simulink model "Quad_model"  (R2024b)
settings: Solver=VariableStepAuto  StartTime=0.0  StopTime=50  RelTol=1e-3
model workspace (MATLAB code in the model file):
  | % Quadcopter parameters
  | m = 1.1;            % Mass [kg]
  | ixx = 8.95e-03;     % Moment of inertia (x-axis) [kg.m^2]
  | iyy = 8.95e-03;     % Moment of inertia (y-axis) [kg.m^2]
  | izz = 0.0165;       % Moment of inertia (z-axis) [kg.m^2]
  | g = 9.81;           % Gravitational acceleration [m/s^2]
  | b = 9.60e-06;       % Thrust coefficient [Ns^2/rad^2]
  | d = 1.24e-07;       % Drag coefficient [Ns^2/rad^2]
  | L = 0.25;           % Arm length [m] (converted from 2.50E-01)
  | I = [ixx, 0, 0;
  |     0, iyy, 0;
  |     0, 0, izz];       % the stifness matrix
  | allocation_matrix_1 = [0, 0.5, 0.25, 0.25;
  |                        -0.5, 0, -0.25, 0.25;
  |                         0, -0.5, 0.25, 0.25;
  |                         0.5, 0, -0.25, 0.25];
  | % Compute pseudo-inverse
  | B = [0, -b*L, 0, b*L;
  |      b*L, 0, -b*L, 0;
  |      d, -d, d, -d;
  |      b, b, b, b];
  | A0 = pinv(B);
  | 
  | % Scale columns by max absolute value
  | A_scaled = zeros(size(A0));
  | for j = 1:size(A0, 2)
  |     col = A0(:, j);
  |     max_abs = max(abs(col));
  |     A_scaled(:, j) = col / max_abs;
  | end
  | allocation_matrix_2 = A_scaled;
  | Kp_h = 30;
  | Kd_h = 89;
  | Kp_yaw = 304;
  | Kd_yaw = 322.8;
  | Kp_th = 25;
  | Kd_th = 15;
  | Kp_x = 0.025;
  | Kd_x = 0.08;
  | Kp_ph = 7.715;
  | Kd_ph = 6.268;
  | Kp_y = 2.3054;
  | Kd_y = 0.5476;
undefined symbols (not defined in the file or in its folder): Sim3dSensor
libraries: aerolibanim x1, sim3dcameralib x1, sim3dlib x1, uavsim3dlib x1, shared6dof x1, SignalEditorBlockLib x1
settings Model: Creator=Ahmed  LastModifiedBy=Ahmed
settings OptimizationCC: DefaultParameterBehavior=Inlined  UseDivisionForNetSlopeComputation=on  GainParamInheritBuiltInType=on  UseFloatMulNetSlope=on  InlineInvariantSignals=on  PassReuseOutputArgsAs=Individual arguments  ZeroExternalMemoryAtStartup=off  ZeroInternalMemoryAtStartup=off  NoFixptDivByZeroProtection=on  EfficientFloat2IntCast=on  LifeSpan=1  OptimizeBlockOrder=speed  DifferentSizesBufferReuse=on  EfficientTunableParamExpr=on
settings DebuggingCC: ParameterTunabilityLossMsg=error
settings HardwareCC: ProdBitPerInt=16  ProdBitPerPointer=16  ProdBitPerSizeT=16  ProdBitPerPtrDiffT=16  ProdLargestAtomicFloat=None  ProdWordSize=8  ProdLongLongMode=on  ProdHWDeviceType=Atmel->AVR
settings SFSimCC: MATLABDynamicMemAlloc=off
settings RTWCC: Description=Embedded Coder  SystemTargetFile=ert.tlc  TemplateMakefile=ert_default_tmf
settings CodeAppCC: ForceParamTrailComments=on  IgnoreCustomStorageClasses=off  OperatorAnnotations=on  SimulinkDataObjDesc=on  SFDataObjDesc=on  CustomSymbolStrGlobalVar=rt$N$M  CustomSymbolStrType=$N$M  CustomSymbolStrFcn=$N$M$F  CustomSymbolStrMacro=$N$M  InsertBlockDesc=on
settings ERTTargetCC: TargetLangStandard=C99 (ISO)  GenerateSampleERTMain=on  IncludeMdlTerminateFcn=off  CombineSignalStateStructs=on  SupportComplex=off  SupportContinuousTime=on  ERTCustomFileTemplate=example_file_process.tlc  ERTFilePackagingFormat=CompactWithDataFile

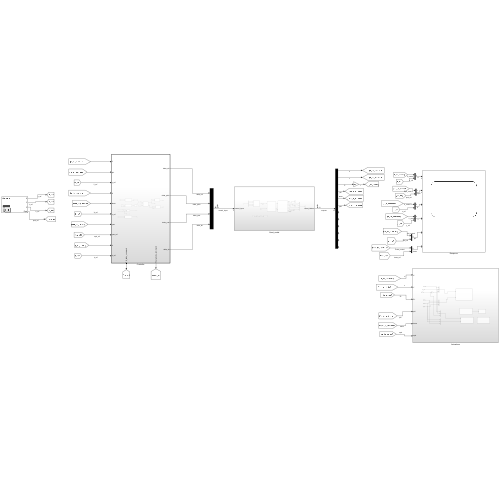
[thumbnail: Simulink's stored preview of the top-level diagram]
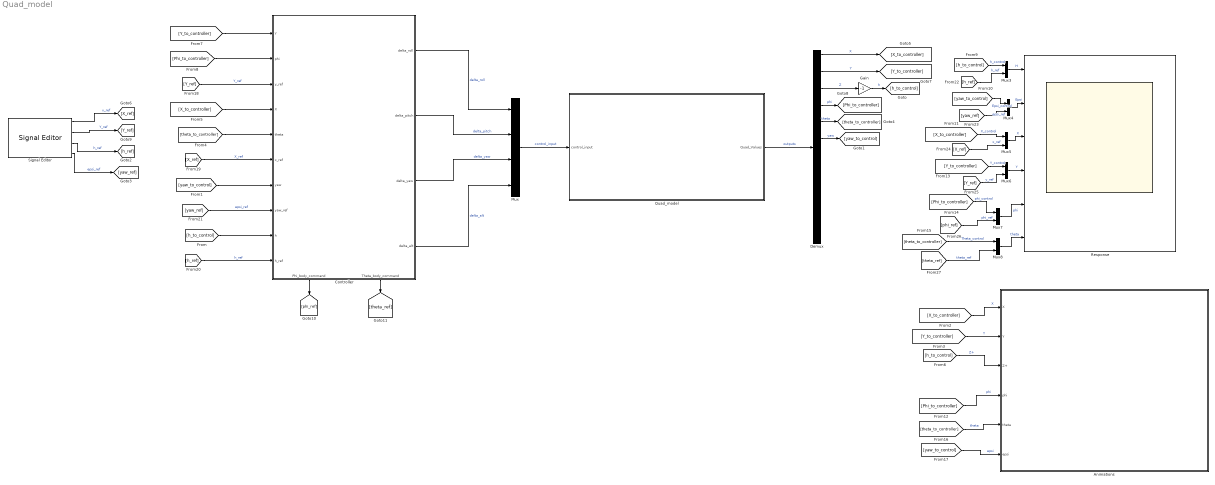
== system Quad_model ==
  Animations : Subsystem
  Controller : Subsystem  TreatAsAtomicUnit=on
      settings: PortSchema="{\"entries\":[{\"content\":{\"sides\":[{\"content\":{\"connectorIds\":[\"In1\",\"In2\",\"In3\",\"In4\",\"In5\",\"In6\",\"In7\",\"In8\",\"In9\",\"In10\"]},\"type\":\"ConnectorPlacement.EquallySpacedRectSide\",\"uuid\":\"5b1a1bc9-4631-4717-aeb0-6531b2b45aea\"},{\"content\":{\"connectorIds\":[\"Out1\",\"Out2\",\"Out3\",\"Out4\"],\"side\":\"RIGHT\"},\"type\":\"ConnectorPlacement.EquallySpacedRectSide\",\"uuid\":\"0754e4a4-abf6-45ed-90c9-fc50fa6a46ef\"},{\"content\":{\"side\":\"TOP\"},\"type\":\"ConnectorPlacement.EquallySpacedRectSide\",\"uuid\":\"f7af2214-f7d2-4adb-8837-c416b6f19e7d\"},{\"content\":{\"connectorIds\":[\"Out5\",\"Out6\"],\"side\":\"BOTTOM\"},\"type\":\"ConnectorPlacement.EquallySpacedRectSide\",\"uuid\":\"41ff5c84-f9d0-4d11-9596-3e8ce6e27fcd\"}]},\"type\":\"ConnectorPlacement.EquallySpacedConnector\",\"uuid\":\"ba43071a-c68b-4035-b336-033c6f17206d\"}],\"packageUris\":[\"http://schema.mathworks.com/mf0/Connector/R2020b\"],\"version\":\"1.0\"}"
  Demux : Demux  Outputs=12
  Gain : Gain  Gain=-1
  Mux : Mux
  Mux{3..8} (6 alike) : Mux  Inputs=2
  Quad_model : Subsystem
  Response : Scope  NumInputPorts=6
  Signal Editor : SignalEditorBlockLib/Signal Editor  FileName=Quad_path.mat  ActiveScenario=Scenario_1  ActiveSignal=X  IsBus=off  OutputBusObjectStr=Bus: BusObject  SampleTime=0  Interpolate=off  ZeroCross=off  OutputAfterFinalValue=Setting to zero  Unit=inherit  PreserveSignalName=on  ApplySigPropsToAllScenarios=on  ApplySigPropsToAllSignals=off
  wires:
  Mux/1 -> Quad_model/1(control_input)  "control_input"
  Quad_model/1(Quad_Values) -> Demux/1  "outputs"
  Controller/1(delta_roll) -> Mux/1  "delta_roll"
  Demux/3 -> Gain/1  "Z"
  Gain/1 -> [h_to_control]  "h"
  [h_ref] -> Controller/10(h_ref)  "h_ref"
  [yaw_ref] -> Controller/8(yaw_ref)  "epsi_ref"
  Demux/6 -> [yaw_to_control]  "yaw"
  [yaw_to_control] -> Controller/7(yaw)
  [h_to_control] -> Controller/9(h)
  Controller/4(delta_alt) -> Mux/4  "delta_alt"
  Controller/3(delta_yaw) -> Mux/3  "delta_yaw"
  Demux/5 -> [theta_to_controller]  "theta"
  [theta_to_controller] -> Controller/5(theta)
  [X_ref] -> Controller/6(x_ref)  "X_ref"
  [X_to_controller] -> Controller/4(X)
  Demux/1 -> [X_to_controller]  "X"
  Controller/2(delta_pitch) -> Mux/2  "delta_pitch"
  Demux/2 -> [Y_to_controller]  "Y"
  [Y_to_controller] -> Controller/1(Y)
  Demux/4 -> [Phi_to_controller]  "phi"
  [Phi_to_controller] -> Controller/2(phi)
  [Y_ref] -> Controller/3(y_ref)  "Y_ref"
  [h_to_control] -> Mux3/1  "h_control"
  [yaw_to_control] -> Mux4/1  "Epsi_control"
  [X_to_controller] -> Mux5/1  "X_control"
  [Y_to_controller] -> Mux6/1  "Y_control"
  [Phi_to_controller] -> Mux7/1  "phi_control"
  [theta_to_controller] -> Mux8/1  "Theta_control"
  Signal Editor/1 -> [X_ref]  "x_ref"
  Signal Editor/2 -> [Y_ref]  "Y_ref"
  Signal Editor/3 -> [h_ref]  "h_ref"
  Signal Editor/4 -> [yaw_ref]  "epsi_ref"
  [h_ref] -> Mux3/2  "h_ref"
  Mux3/1 -> Response/1  "H"
  [yaw_ref] -> Mux4/2  "epsi_ref"
  Mux4/1 -> Response/2  "Epsi"
  Mux5/1 -> Response/3  "X"
  [X_ref] -> Mux5/2  "x_ref"
  Mux6/1 -> Response/4  "Y"
  [Y_ref] -> Mux6/2  "y_ref"
  Controller/5(Phi_body_command) -> [phi_ref]
  Controller/6(Theta_body_command) -> [theta_ref]
  [phi_ref] -> Mux7/2  "phi_ref"
  Mux7/1 -> Response/5  "phi"
  Mux8/1 -> Response/6  "theta"
  [theta_ref] -> Mux8/2  "theta_ref"
  [X_to_controller] -> Animations/1(X)  "X"
  [Y_to_controller] -> Animations/2(Y)  "Y"
  [h_to_control] -> Animations/3(Z+)  "Z+"
  [Phi_to_controller] -> Animations/4(phi)  "phi"
  [theta_to_controller] -> Animations/5(theta)  "theta"
  [yaw_to_control] -> Animations/6(epsi)  "epsi"

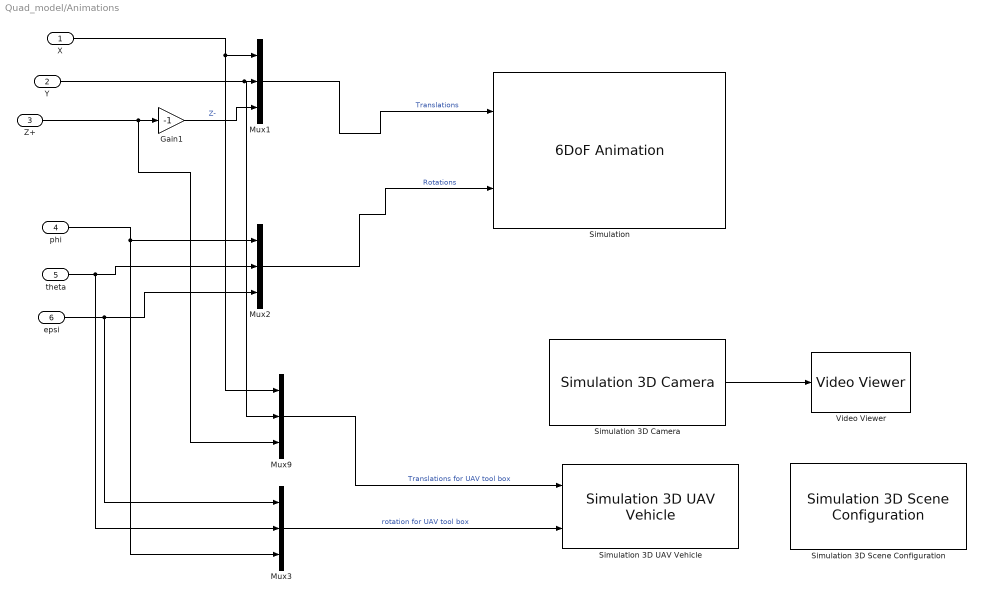
== system Quad_model/Animations ==
  X : Inport
  Y : Inport  Port=2
  Z+ : Inport  Port=3
  phi : Inport  Port=4
  theta : Inport  Port=5
  epsi : Inport  Port=6
  Gain1 : Gain  Gain=-1
  Mux{1..3,9} (4 alike) : Mux  Inputs=3
  Simulation : aerolibanim/6DoF Animation  u1=[-8 8 -8 8 -6 0]  u2=0.1  u3=1.0  u4=[0 0 0]  u5=Fixed position  u6=[20 50 -20]  u7=10  u8=on
  Simulation 3D Camera : sim3dcameralib/Simulation 3D Camera  Priority=1  sensorTag=Sim3dSensor�  sensorId=2  sensorName=Sim3dSensor�  vehTagList={'Scene Origin';'SimulinkVehicle1'}  vehTag=SimulinkVehicle1  mountLoc=Origin  offsetFlag=on  tmountOffset=[0.1, 0, 0]  extTmount=off  rmountOffset=[0, 0, 0]  extRmount=off  FocalLength=[1109, 1109]  OpticalCenter=[640, 360]  ImageSize=[720, 1280]  RadialDistortion=[0, 0]  TangentialDistortion=[0, 0]  SensorSkew=0  DepthOutportEnabled=off  SemanticOutportEnabled=off  TransformOutportEnabled=off  SampleTime=-1  mountPoint=[0.1 0 0]  mountOrientation=[0 0 0]  aMode=4  ID=2
      settings: LibrarySourceBlock=uavsim3dlib/Simulation 3D Camera
  Simulation 3D Scene Configuration : sim3dlib/Simulation 3D Scene Configuration  Priority=0  ProjectFormat=Default Scenes  SceneDesc=US city block  ProjectName=C:\Program Files\MATLAB\R2024b\toolbox\shared\sim3d_projects\automotive_project_windows\UE\WindowsNoEditor\VehicleSimulation.exe  ScenePath=/Game/Maps/USCityBlock  EnableOpenDRIVE=off  vehTagList={'Custom';'Scene Origin';'SimulinkVehicle1'}  vehTag=SimulinkVehicle1  FreeCameraInitialTranslation=[0, 0, 0]  FreeCameraDefaultInitialTranslation=[-6, 0, 2]  FreeCameraInitialRotation=[0, 0, 0]  FreeCameraDefaultInitialRotation=[0, -15, 0]  OpVisEn=off  Ts=0.1  EnableWindow=on  EnableRemoteAccess=off  EnableWeather=off  SunAzimuth=90  SunAltitude=40.0  EnableGeospatialSun=off  Latitude=0  Longitude=0  Date=2023-01-01  Time=10:30:00  GeoTimeZone=-5.0  SunDaylightSaving=off  wind=1  clouds=10  EnableVolumetricClouds=off  CloudCoverage=0  CloudAltitude=6  fog=0  rain=0  RaindropsEffect=off  SnowDensity=0  EnableGeospatial=off  UseTrueOrigin=off  OriginHeight=200  OriginLatitude=40.744652  OriginLongitude=-73.988864  MapStyle=Aerial  AdditionalAssetIDs=[]  UseAdvancedSunSky=off  SolarTime=11  TimeZone=-5  Day=21  Month=9  Year=2022  UseDaylightSavingTime=on  DSTStartDay=10  DSTStartMonth=3  DSTEndDay=3  DSTEndMonth=11  DSTSwitchHour=2  sensorTag=MainCamera1  sensorId=1  sensorName=MainCamera1  mountLoc=Origin  offsetFlag=off  tmountOffset=[0, 0, 0]  rmountOffset=[0, 0, 0]  HorizontalResolution=1280  VerticalResolution=720  HorizontalFOV=60  mountPoint=[0 0 0]  mountOrientation=[0 0 0]  aMode=4  ID=1  GeoTrigger=Inactive
      settings: LibrarySourceBlock=uavsim3dlib/Simulation 3D Scene Configuration
  Simulation 3D UAV Vehicle : uavsim3dlib/Simulation 3D UAV Vehicle  Priority=-1  Mesh=Quadrotor  MeshPath=/MathWorksUAVContent/UAVs/HexaRotorUAV/HexaRotor.HexaRotor  Color=Black  ActorName=SimulinkVehicle1  UseGlobalFrame=off  InitialTranslation=[0 0 0]  InitialRotation=[0 0 0]  InitialTranslationGlobal=[0 0 0]  InitialGeoOrigin=[0 0 0]  InitialRotationGlobal=[0 0 0]  SampleTime=0.1  ActorType=SimulinkVehicle  ID=1  aMode=4  ActorTag=SimulinkVehicle1
  Video Viewer : VideoViewer  FigPos=[1107.4 562.8 417.6 304]
  wires:
  Mux2/1 -> Simulation/2  "Rotations"
  X/1 -> Mux9/1, Mux1/1
  Gain1/1 -> Mux1/3  "Z-"
  Z+/1 -> Mux9/3, Gain1/1
  Mux9/1 -> Simulation 3D UAV Vehicle/1  "Translations for UAV tool box"
  Mux1/1 -> Simulation/1  "Translations"
  Y/1 -> Mux9/2, Mux1/2
  phi/1 -> Mux3/3, Mux2/1
  theta/1 -> Mux3/2, Mux2/2
  epsi/1 -> Mux3/1, Mux2/3
  Mux3/1 -> Simulation 3D UAV Vehicle/2  "rotation for UAV tool box"
  Simulation 3D Camera/1 -> Video Viewer/1

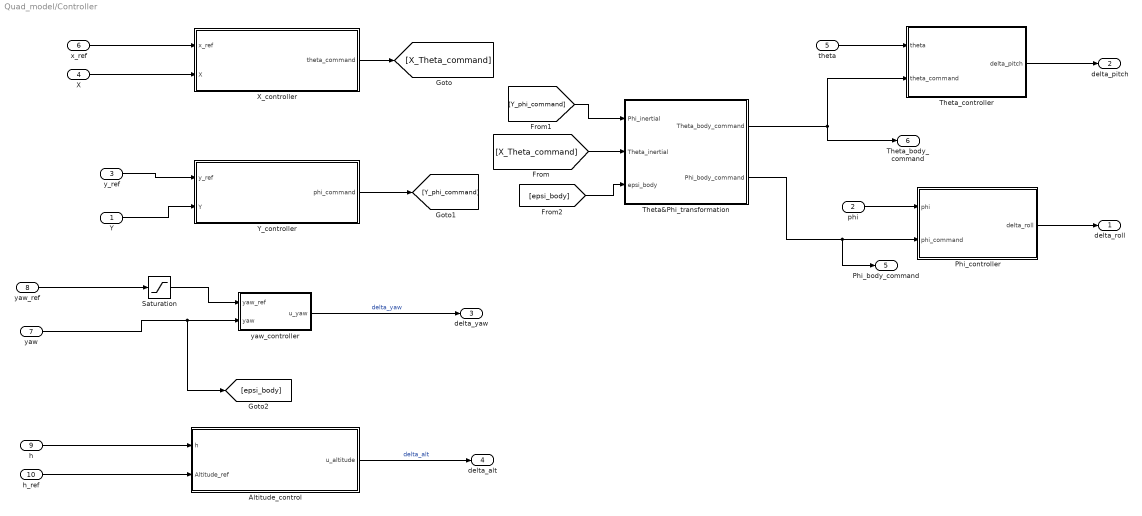
== system Quad_model/Controller ==
  Y : Inport
  phi : Inport  Port=2
  y_ref : Inport  Port=3
  X : Inport  Port=4
  theta : Inport  Port=5
  x_ref : Inport  Port=6
  yaw : Inport  Port=7
  yaw_ref : Inport  Port=8
  h : Inport  Port=9
  h_ref : Inport  Port=10
  Altitude_control : Subsystem
  Phi_controller : Subsystem
  Saturation : Saturate  UpperLimit=3  LowerLimit=-3
  Theta&Phi_transformation : Subsystem
  Theta_controller : Subsystem
  X_controller : Subsystem
  Y_controller : Subsystem
  yaw_controller : Subsystem
  delta_roll : Outport
  delta_pitch : Outport  Port=2
  delta_yaw : Outport  Port=3
  delta_alt : Outport  Port=4
  Phi_body_command : Outport  Port=5
  Theta_body_command : Outport  Port=6
  wires:
  yaw_controller/1(u_yaw) -> delta_yaw/1  "delta_yaw"
  h_ref/1 -> Altitude_control/2(Altitude_ref)
  h/1 -> Altitude_control/1(h)
  yaw_ref/1 -> Saturation/1
  Altitude_control/1(u_altitude) -> delta_alt/1  "delta_alt"
  yaw/1 -> [epsi_body], yaw_controller/2(yaw)
  Theta_controller/1(delta_pitch) -> delta_pitch/1
  Theta&Phi_transformation/1(Theta_body_command) -> Theta_controller/2(theta_command), Theta_body_command/1
  X_controller/1(theta_command) -> [X_Theta_command]
  x_ref/1 -> X_controller/1(x_ref)
  X/1 -> X_controller/2(X)
  Phi_controller/1(delta_roll) -> delta_roll/1
  Theta&Phi_transformation/2(Phi_body_command) -> Phi_body_command/1, Phi_controller/2(phi_command)
  Y_controller/1(phi_command) -> [Y_phi_command]
  y_ref/1 -> Y_controller/1(y_ref)
  Y/1 -> Y_controller/2(Y)
  phi/1 -> Phi_controller/1(phi)
  theta/1 -> Theta_controller/1(theta)
  [X_Theta_command] -> Theta&Phi_transformation/2(Theta_inertial)
  [Y_phi_command] -> Theta&Phi_transformation/1(Phi_inertial)
  [epsi_body] -> Theta&Phi_transformation/3(epsi_body)
  Saturation/1 -> yaw_controller/1(yaw_ref)

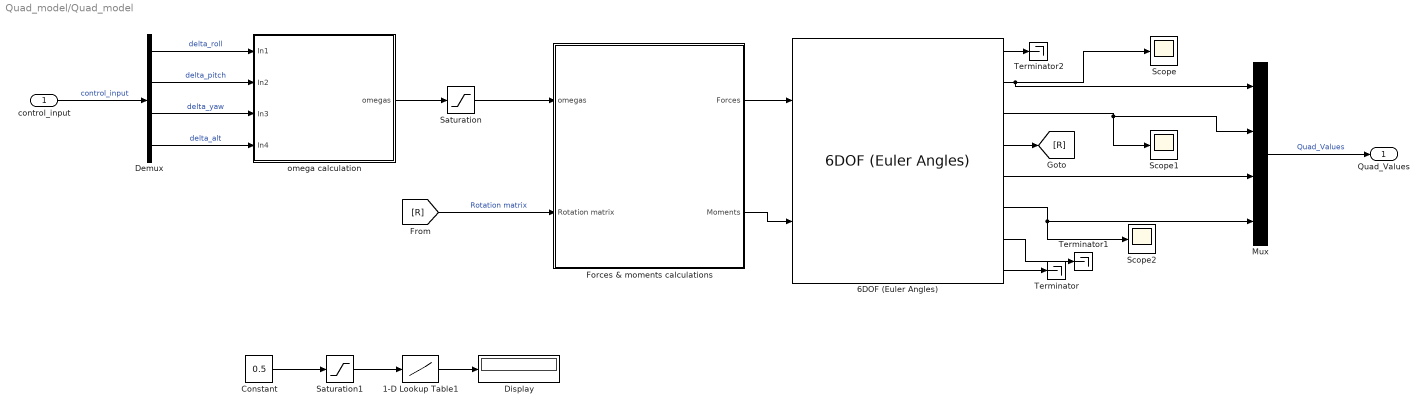
== system Quad_model/Quad_model ==
  control_input : Inport  OutDataTypeStr=double  PortDimensions=4
  1-D Lookup Table1 : Lookup_n-D  NumberOfTableDimensions=1  BreakpointsForDimension1=[-1,1]  Table=[0,sqrt(2*m*g/(4*b))]  InternalRulePriority=Speed  RndMeth=Simplest
  6DOF (Euler Angles) : shared6dof/6DOF (Euler Angles)  units=Metric (MKS)  mtype=Fixed  rep=Euler Angles  xme_0=[0 0 -1]  Vm_0=[0 0 0]  eul_0=[0 0 0]  pm_0=[0 0 0]  mass_0=m  mass_e=0.5  mass_f=2.0  inertia=I  inertia_e=eye(3)  inertia_f=2*eye(3)  k_quat=1.0  vre_flag=on  abi_flag=off  aMode=0  xme_statename=''  Vm_statename=''  eul_statename=''  quat_statename=''  pm_statename=''  mass_statename=''
  Constant : Constant  Value=0.5
  Demux : Demux
  Display : Display
  Forces & moments calculations : Subsystem
  Mux : Mux
  Saturation : Saturate  UpperLimit=sqrt(2*m*g/(4*b))  LowerLimit=0
  Saturation1 : Saturate  UpperLimit=1  LowerLimit=-1
  Scope : Scope
  Scope1 : Scope
  Scope2 : Scope
  Terminator : Terminator
  Terminator1 : Terminator
  Terminator2 : Terminator
  omega calculation : Subsystem
  Quad_Values : Outport  OutDataTypeStr=double  PortDimensions=12  SampleTime=0
  wires:
  6DOF (Euler Angles)/5 -> Mux/3
  6DOF (Euler Angles)/6 -> Scope2/1, Mux/4
  control_input/1 -> Demux/1  "control_input"
  6DOF (Euler Angles)/7 -> Terminator1/1
  Saturation1/1 -> 1-D Lookup Table1/1
  omega calculation/1(omegas) -> Saturation/1
  Demux/2 -> omega calculation/2(In2)  "delta_pitch"
  6DOF (Euler Angles)/2 -> Mux/1, Scope/1
  Saturation/1 -> Forces & moments calculations/1(omegas)
  [R] -> Forces & moments calculations/2(Rotation matrix)  "Rotation matrix"
  6DOF (Euler Angles)/4 -> [R]
  Forces & moments calculations/1(Forces) -> 6DOF (Euler Angles)/1
  1-D Lookup Table1/1 -> Display/1
  6DOF (Euler Angles)/1 -> Terminator2/1
  Constant/1 -> Saturation1/1
  Demux/1 -> omega calculation/1(In1)  "delta_roll"
  Demux/3 -> omega calculation/3(In3)  "delta_yaw"
  Demux/4 -> omega calculation/4(In4)  "delta_alt"
  6DOF (Euler Angles)/8 -> Terminator/1
  Mux/1 -> Quad_Values/1  "Quad_Values"
  Forces & moments calculations/2(Moments) -> 6DOF (Euler Angles)/2
  6DOF (Euler Angles)/3 -> Scope1/1, Mux/2

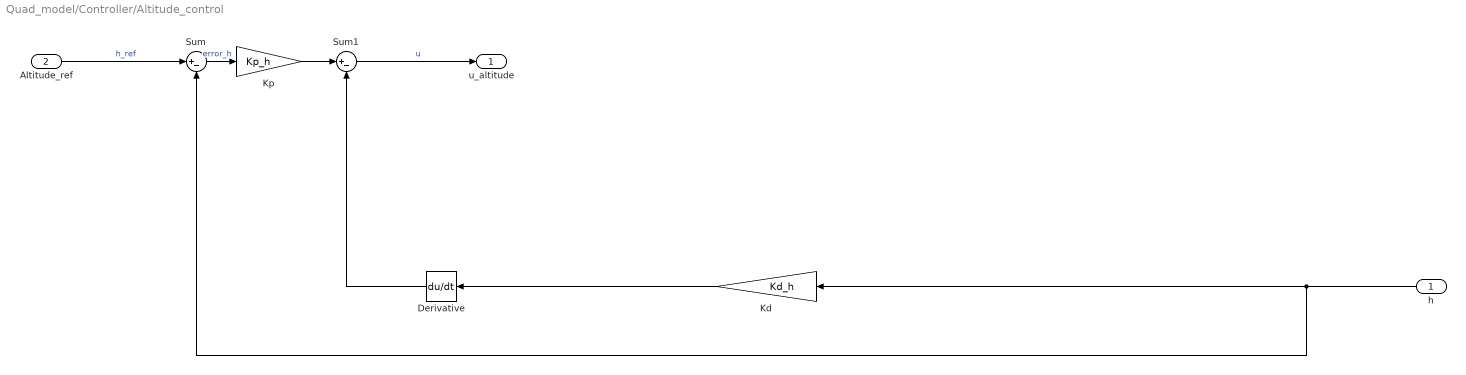
== system Quad_model/Controller/Altitude_control ==
  h : Inport
  Altitude_ref : Inport  Port=2
  Derivative : Derivative
  Kd : Gain  Gain=Kd_h
  Kp : Gain  Gain=Kp_h
  Sum : Sum  Inputs=|+-
  Sum1 : Sum  Inputs=|+-
  u_altitude : Outport
  wires:
  Sum/1 -> Kp/1  "error_h"
  Altitude_ref/1 -> Sum/1  "h_ref"
  Kd/1 -> Derivative/1
  Kp/1 -> Sum1/1
  h/1 -> Kd/1, Sum/2
  Derivative/1 -> Sum1/2
  Sum1/1 -> u_altitude/1  "u"

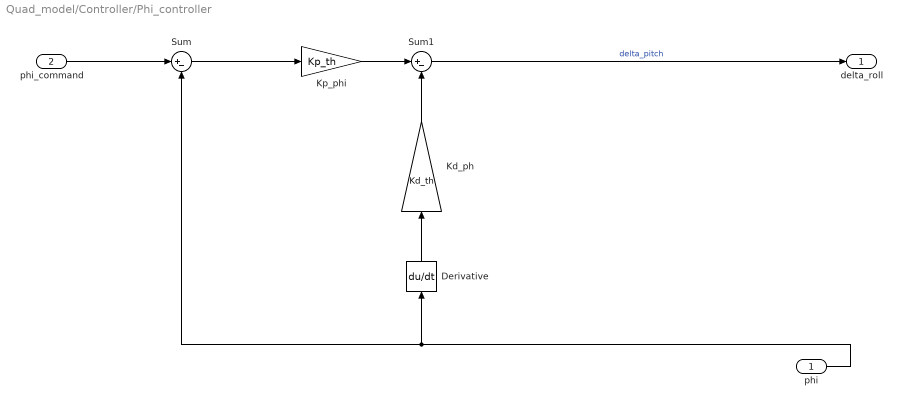
== system Quad_model/Controller/Phi_controller ==
  phi : Inport
  phi_command : Inport  Port=2
  Derivative : Derivative
  Kd_ph : Gain  Gain=Kd_th
  Kp_phi : Gain  Gain=Kp_th
  Sum : Sum  Inputs=|+-
  Sum1 : Sum  Inputs=|+-
  delta_roll : Outport
  wires:
  Kp_phi/1 -> Sum1/1
  Sum/1 -> Kp_phi/1
  Kd_ph/1 -> Sum1/2
  phi/1 -> Sum/2, Derivative/1
  phi_command/1 -> Sum/1
  Sum1/1 -> delta_roll/1  "delta_pitch"
  Derivative/1 -> Kd_ph/1

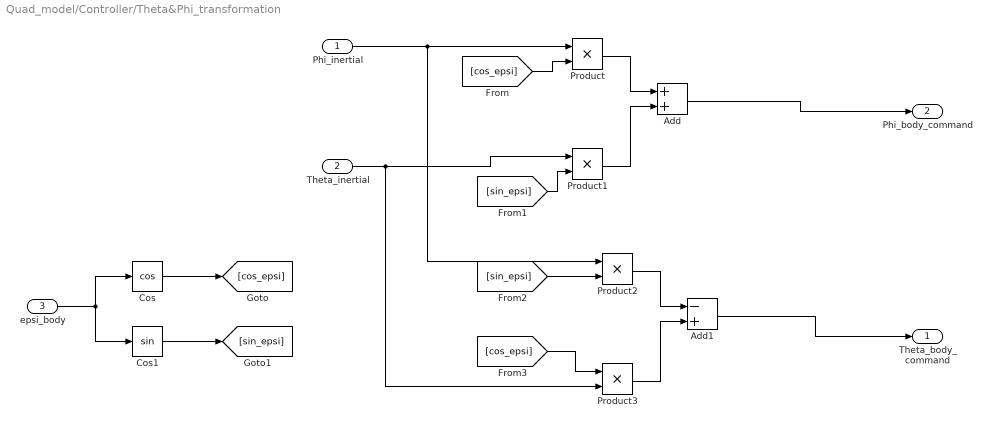
== system Quad_model/Controller/Theta&Phi_transformation ==
  Phi_inertial : Inport
  Theta_inertial : Inport  Port=2
  epsi_body : Inport  Port=3
  Add : Sum
  Add1 : Sum  Inputs=-+
  Cos : Trigonometry  Operator=cos
  Cos1 : Trigonometry
  Product{,1..3} (4 alike) : Product
  Theta_body_command : Outport
  Phi_body_command : Outport  Port=2
  wires:
  Phi_inertial/1 -> Product2/1, Product/1
  epsi_body/1 -> Cos1/1, Cos/1
  Cos/1 -> [cos_epsi]
  Theta_inertial/1 -> Product3/2, Product1/1
  Cos1/1 -> [sin_epsi]
  Product/1 -> Add/1
  Product1/1 -> Add/2
  [cos_epsi] -> Product/2
  [sin_epsi] -> Product1/2
  Add/1 -> Phi_body_command/1
  Product3/1 -> Add1/2
  Product2/1 -> Add1/1
  [sin_epsi] -> Product2/2
  [cos_epsi] -> Product3/1
  Add1/1 -> Theta_body_command/1

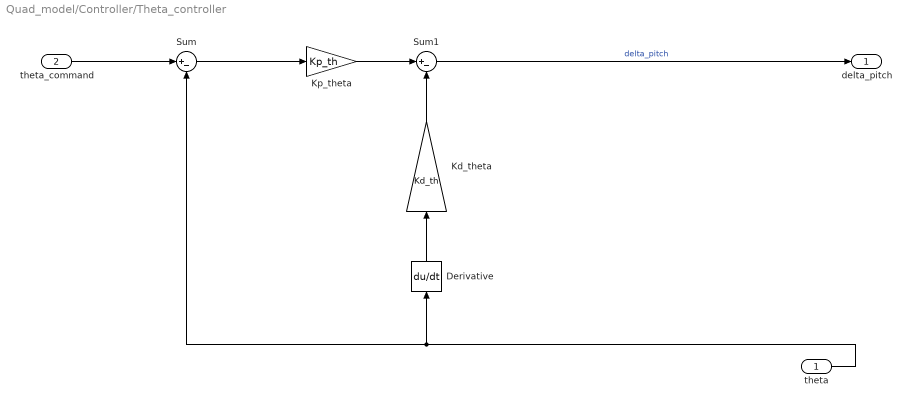
== system Quad_model/Controller/Theta_controller ==
  theta : Inport
  theta_command : Inport  Port=2
  Derivative : Derivative
  Kd_theta : Gain  Gain=Kd_th
  Kp_theta : Gain  Gain=Kp_th
  Sum : Sum  Inputs=|+-
  Sum1 : Sum  Inputs=|+-
  delta_pitch : Outport
  wires:
  Kp_theta/1 -> Sum1/1
  Sum/1 -> Kp_theta/1
  Kd_theta/1 -> Sum1/2
  theta/1 -> Sum/2, Derivative/1
  theta_command/1 -> Sum/1
  Sum1/1 -> delta_pitch/1  "delta_pitch"
  Derivative/1 -> Kd_theta/1

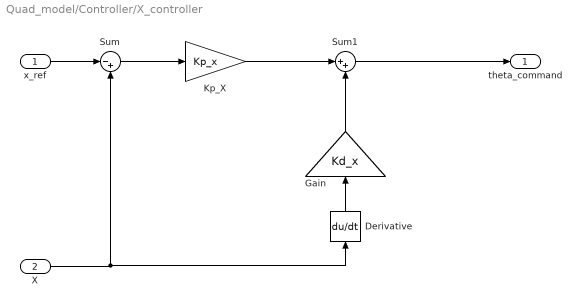
== system Quad_model/Controller/X_controller ==
  x_ref : Inport
  X : Inport  Port=2
  Derivative : Derivative
  Gain : Gain  Gain=Kd_x
  Kp_X : Gain  Gain=Kp_x
  Sum : Sum  Inputs=|-+
  Sum1 : Sum  Inputs=|++
  theta_command : Outport
  wires:
  x_ref/1 -> Sum/1
  X/1 -> Sum/2, Derivative/1
  Sum/1 -> Kp_X/1
  Derivative/1 -> Gain/1
  Kp_X/1 -> Sum1/1
  Gain/1 -> Sum1/2
  Sum1/1 -> theta_command/1

== system Quad_model/Controller/Y_controller ==
  y_ref : Inport
  Y : Inport  Port=2
  Derivative : Derivative
  Kd_y : Gain  Gain=Kd_x
  Kp_y : Gain  Gain=Kp_x
  Sum : Sum  Inputs=|+-
  Sum1 : Sum  Inputs=|+-
  phi_command : Outport
  wires:
  y_ref/1 -> Sum/1
  Y/1 -> Sum/2, Derivative/1
  Sum/1 -> Kp_y/1
  Derivative/1 -> Kd_y/1
  Kp_y/1 -> Sum1/1
  Kd_y/1 -> Sum1/2
  Sum1/1 -> phi_command/1

== system Quad_model/Controller/yaw_controller ==
  yaw_ref : Inport
  yaw : Inport  Port=2
  Derivative : Derivative
  Gain : Gain  Gain=Kp_yaw
  Gain1 : Gain  Gain=Kd_yaw
  Sum : Sum  Inputs=|+-
  Sum1 : Sum  Inputs=|+-
  u_yaw : Outport
  wires:
  Gain/1 -> Sum1/1
  yaw/1 -> Sum/2, Derivative/1
  Gain1/1 -> Sum1/2
  Sum1/1 -> u_yaw/1
  Sum/1 -> Gain/1
  Derivative/1 -> Gain1/1
  yaw_ref/1 -> Sum/1

== system Quad_model/Quad_model/Forces & moments calculations ==
  omegas : Inport
  Rotation matrix : Inport  Port=2
  Forces calculations : Subsystem
  momemnts : Subsystem
  Forces : Outport
  Moments : Outport  Port=2
  wires:
  Forces calculations/1(Forces) -> Forces/1
  Rotation matrix/1 -> Forces calculations/1(Rotation matrix)
  momemnts/1(Moments) -> Moments/1
  omegas/1 -> momemnts/1(omegas), Forces calculations/2(omegas)

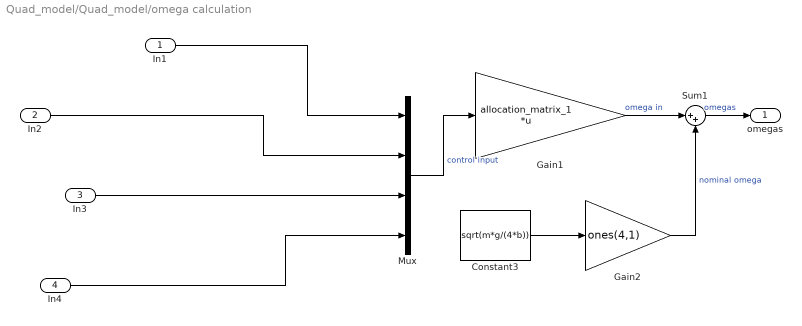
== system Quad_model/Quad_model/omega calculation ==
  In1 : Inport
  In2 : Inport  Port=2
  In3 : Inport  Port=3
  In4 : Inport  Port=4
  Constant3 : Constant  Value=sqrt(m*g/(4*b))  VectorParams1D=off
  Gain1 : Gain  Gain=allocation_matrix_1  Multiplication=Matrix(K*u)
  Gain2 : Gain  Gain=ones(4,1)
  Mux : Mux
  Sum1 : Sum  Inputs=|++
  omegas : Outport
  wires:
  Mux/1 -> Gain1/1  "control input"
  In2/1 -> Mux/2
  Gain1/1 -> Sum1/1  "omega in"
  Constant3/1 -> Gain2/1
  Gain2/1 -> Sum1/2  "nominal omega"
  In3/1 -> Mux/3
  In4/1 -> Mux/4
  In1/1 -> Mux/1
  Sum1/1 -> omegas/1  "omegas"

== system Quad_model/Quad_model/Forces & moments calculations/Forces calculations ==
  Rotation matrix : Inport
  omegas : Inport  Port=2
  External forces : Subsystem
  Gain : Gain  Gain=[0; 0; m*g]  Multiplication=Matrix(u*K)
  Sum : Sum  Inputs=|++
  Forces : Outport
  wires:
  Gain/1 -> Sum/2
  omegas/1 -> External forces/1(omegas)
  External forces/1(thrust component) -> Sum/1
  Rotation matrix/1 -> Gain/1
  Sum/1 -> Forces/1  "forces"

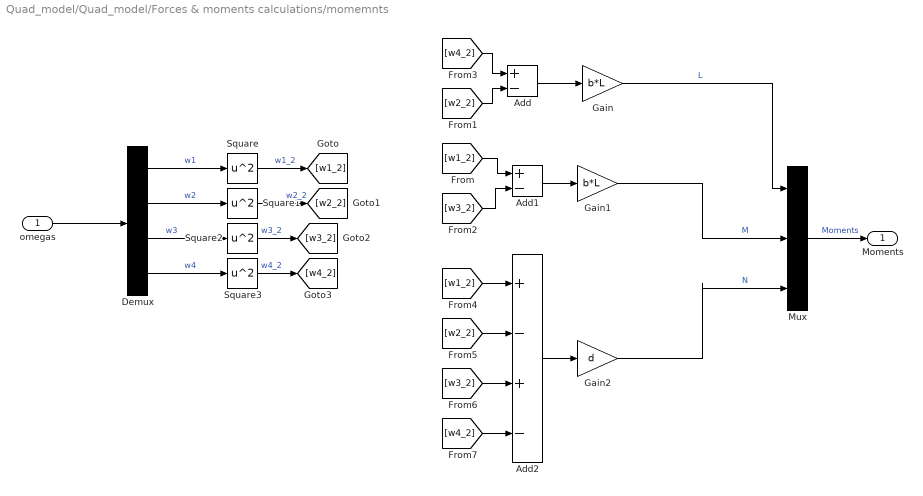
== system Quad_model/Quad_model/Forces & moments calculations/momemnts ==
  omegas : Inport
  Add : Sum  Inputs=+-
  Add1 : Sum  Inputs=+-
  Add2 : Sum  Inputs=+-+-
  Demux : Demux
  Gain : Gain  Gain=b*L
  Gain1 : Gain  Gain=b*L
  Gain2 : Gain  Gain=d
  Mux : Mux  Inputs=3
  Square{,1..3} (4 alike) : Math  Operator=square
  Moments : Outport
  wires:
  Gain2/1 -> Mux/3  "N"
  Gain1/1 -> Mux/2  "M"
  Gain/1 -> Mux/1  "L"
  Mux/1 -> Moments/1  "Moments"
  [w2_2] -> Add2/2
  [w3_2] -> Add2/3
  [w4_2] -> Add2/4
  [w1_2] -> Add2/1
  Add2/1 -> Gain2/1
  [w3_2] -> Add1/2
  [w1_2] -> Add1/1
  Add1/1 -> Gain1/1
  [w2_2] -> Add/2
  [w4_2] -> Add/1
  Add/1 -> Gain/1
  Square/1 -> [w1_2]  "w1_2"
  Square2/1 -> [w3_2]  "w3_2"
  Square3/1 -> [w4_2]  "w4_2"
  Square1/1 -> [w2_2]  "w2_2"
  Demux/4 -> Square3/1  "w4"
  Demux/3 -> Square2/1  "w3"
  Demux/2 -> Square1/1  "w2"
  Demux/1 -> Square/1  "w1"
  omegas/1 -> Demux/1

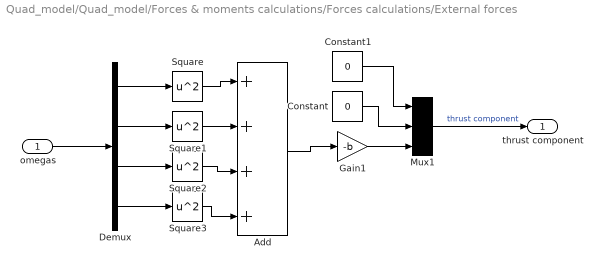
== system Quad_model/Quad_model/Forces & moments calculations/Forces calculations/External forces ==
  omegas : Inport
  Add : Sum  Inputs=++++
  Constant : Constant  Value=0  VectorParams1D=off
  Constant1 : Constant  Value=0  VectorParams1D=off
  Demux : Demux
  Gain1 : Gain  Gain=-b
  Mux1 : Mux  Inputs=3
  Square{,1..3} (4 alike) : Math  Operator=square
  thrust component : Outport
  wires:
  Mux1/1 -> thrust component/1  "thrust component"
  omegas/1 -> Demux/1
  Gain1/1 -> Mux1/3
  Constant/1 -> Mux1/2
  Square2/1 -> Add/3
  Demux/4 -> Square3/1
  Constant1/1 -> Mux1/1
  Demux/2 -> Square1/1
  Demux/1 -> Square/1
  Square1/1 -> Add/2
  Square/1 -> Add/1
  Demux/3 -> Square2/1
  Square3/1 -> Add/4
  Add/1 -> Gain1/1
